simulink model "LookupTableND_evenSpacing_vector_inputs"  (R2017b)
settings: Solver=FixedStepDiscrete  StartTime=0.0  StopTime=10.0  FixedStep=0.200000  RelTol=1e-3  EnableMultiTasking=on
settings Model: Creator=hbourbou  LastModifiedBy=hbourbou
settings DataIOCC: LimitDataPoints=on  SaveFormat=StructureWithTime
settings OptimizationCC: LifeSpan=inf
settings DebuggingCC: SFUnexpectedBacktrackingDiag=warning  SFNoUnconditionalDefaultTransitionDiag=warning  SFExecutionAtInitializationDiag=none
settings HardwareCC: ProdBitPerSizeT=32  ProdBitPerPtrDiffT=32  ProdWordSize=32  ProdHWDeviceType=Specified
settings ModelReferenceCC: PropagateSignalLabelsOutOfModel=off
settings CodeAppCC: StateflowObjectComments=on
settings GRTTargetCC: TargetLangStandard=C89/C90 (ANSI)
settings ConfigComp: CovMetricSettings=dw  CovHtmlReporting=on  CovSaveCumulativeToWorkspaceVar=on  CovSaveSingleToWorkspaceVar=on  CovExternalEMLEnable=off

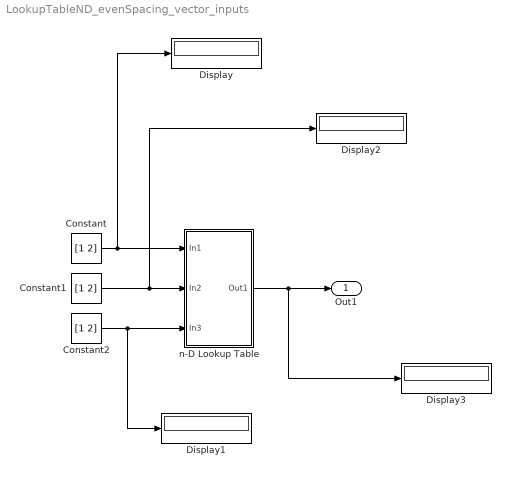
== system LookupTableND_evenSpacing_vector_inputs ==
  Constant : Constant  Value=[1 2]
  Constant1 : Constant  Value=[1 2]
  Constant2 : Constant  Value=[1 2]
  Display{,1..3} (4 alike) : Display
  n-D Lookup Table : Subsystem  Description=Replaced Block  mask(Replaced Block){}
      mask help: This block has been replaced with an empty subsystem because it used functionality that is unavailable in Simulink R2015a.
      mask Display: fprintf('Replaced: %s\n','Lookup_n-D')
  Out1 : Outport
  wires:
  Constant/1 -> Display/1, n-D Lookup Table/1(In1)
  Constant1/1 -> Display2/1, n-D Lookup Table/2(In2)
  Constant2/1 -> Display1/1, n-D Lookup Table/3(In3)
  n-D Lookup Table/1(Out1) -> Display3/1, Out1/1

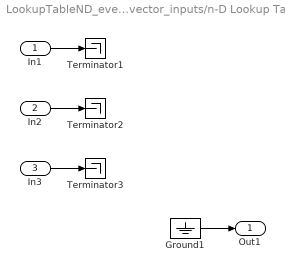
== system LookupTableND_evenSpacing_vector_inputs/n-D Lookup Table ==
  In1 : Inport
  In2 : Inport  Port=2
  In3 : Inport  Port=3
  Ground1 : Ground
  Terminator1 : Terminator
  Terminator2 : Terminator
  Terminator3 : Terminator
  Out1 : Outport
  wires:
  Ground1/1 -> Out1/1
  In3/1 -> Terminator3/1
  In2/1 -> Terminator2/1
  In1/1 -> Terminator1/1
